simulink model "model"  (R2015a)
settings: Solver=ode45  StartTime=0.0  RelTol=1e-3
values from neighbouring files (symbols this model uses):
  A = [-31.31 0 -2.833e4 2; 0 -10.25 8001 0; 1 -1 0 0; 0 0 0 -100]    [Copy_of_UIE_tracking_main.m]    (also in UIE_main.m = [0 0 1 0; 0 0 0 1; -3 1 -0.4 0.1; 1 -1 0.1 -0.1]; UIE_tracking_main.m = [0 0 1 0; 0 0 0 1; -3 1 -0.4 0.1; 1 -1 0.1 -0.1])
  Af = [-100 0; 0 -100]    [Copy_of_UIE_tracking_main.m]    (also in UIE_main.m; UIE_tracking_main.m)
  B = [28.06 0 0 1; 0 28.06 0 1]'    [Copy_of_UIE_tracking_main.m]    (also in UIE_main.m = [0 0; 0 0; 1 0; 0 1]; UIE_tracking_main.m = [0 0; 0 0; 1 0; 0 1])
  Bd = B    [Copy_of_UIE_tracking_main.m]    (also in UIE_main.m = [0 0 0; 0 0 0; 1 0.5 0.75; 0.5 1 0.75]; UIE_tracking_main.m)
  Bf = [8 0; 0 8]    [Copy_of_UIE_tracking_main.m]    (also in UIE_main.m; UIE_tracking_main.m)
  C = [1 0 0 0;1 0 30 0]    [Copy_of_UIE_tracking_main.m]    (also in UIE_main.m = [1 0 0 0; 0 1 0 0]; UIE_tracking_main.m = [1 0 0 0; 0 1 0 0])
  Cf = [12.5 0; 0 12.5]    [Copy_of_UIE_tracking_main.m]    (also in UIE_main.m; UIE_tracking_main.m)
  Ec = -inv(Rc)*B'*inv(A - B*Kc)'*C'*Qc    [Copy_of_UIE_tracking_main.m]    (also in UIE_main.m; UIE_tracking_main.m)
  Kc = lqr(A + Hc*eye(n), B, C'*Qc*C, Rc)    [Copy_of_UIE_tracking_main.m]    (also in UIE_main.m; UIE_tracking_main.m)
  Kd = pinv(B)*Lt    [Copy_of_UIE_tracking_main.m]    (also in UIE_main.m; UIE_tracking_main.m)
  L = lqr(A'+H*eye(n), C', Qo, Ro)'    [Copy_of_UIE_tracking_main.m]    (also in UIE_main.m; UIE_tracking_main.m)
  Tf = 1e-3    (= 0.001)    [Copy_of_UIE_tracking_main.m]    (also in UIE_main.m; UIE_tracking_main.m)
  x_ini = [0 0 0 0]    [Copy_of_UIE_tracking_main.m]    (also in UIE_main.m = [0 1 0 0]; UIE_tracking_main.m)
  xo_ini = [0 0 0 0]    [Copy_of_UIE_tracking_main.m]    (also in UIE_main.m = [0 1 0 0]; UIE_tracking_main.m)
settings Model: CovSFcnEnable=off  Creator=123  LastModifiedBy=Elca
settings DebuggingCC: UnconnectedInputMsg=none  UnconnectedOutputMsg=none

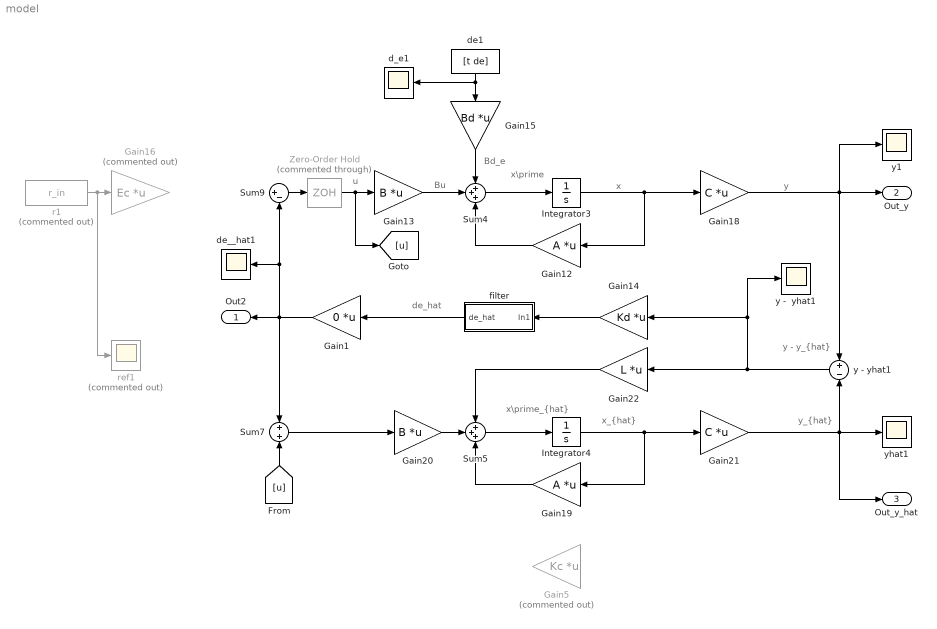
== system model ==
  note: de_hat
  note: Bd_e
  note: Bu
  note: y - y_{hat}
  note: x\prime
  note: x\prime_{hat}
  note: x_{hat}
  note: y_{hat}
  note: x
  note: y
  note: u
  Gain1 : Gain  Gain=0  Multiplication=Matrix(K*u)
  Gain12 : Gain  Gain=A  Multiplication=Matrix(K*u)
  Gain13 : Gain  Gain=B  Multiplication=Matrix(K*u)
  Gain14 : Gain  Gain=Kd  Multiplication=Matrix(K*u)
  Gain15 : Gain  Gain=Bd  Multiplication=Matrix(K*u)
  Gain16 : Gain  Commented=on  Gain=Ec  Multiplication=Matrix(K*u)
  Gain18 : Gain  Gain=C  Multiplication=Matrix(K*u)
  Gain19 : Gain  Gain=A  Multiplication=Matrix(K*u)
  Gain20 : Gain  Gain=B  Multiplication=Matrix(K*u)
  Gain21 : Gain  Gain=C  Multiplication=Matrix(K*u)
  Gain22 : Gain  Gain=L  Multiplication=Matrix(K*u)
  Gain5 : Gain  Commented=on  Gain=Kc  Multiplication=Matrix(K*u)
  Integrator3 : Integrator  InitialCondition=x_ini
  Integrator4 : Integrator  InitialCondition=xo_ini
  Sum4 : Sum  Inputs=+++
  Sum5 : Sum  Inputs=+++
  Sum7 : Sum  Inputs=+|+
  Sum9 : Sum  Inputs=|+-
  Zero-Order Hold : ZeroOrderHold  Commented=through  SampleTime=Tf
  d_e1 : Scope
      settings: TickLabels=on  ShowLegends=on  SaveName=ScopeData6  ScrollMode=on
  de1 : FromWorkspace  VariableName=[t de]  SampleTime=0
  de__hat1 : Scope
      settings: TickLabels=on  ShowLegends=on  SaveName=ScopeData7  ScrollMode=on
  filter : Subsystem
  r1 : FromWorkspace  Commented=on  VariableName=r_in  SampleTime=Tf
  ref1 : Scope  Commented=on
      settings: TickLabels=on  YMin=0  YMax=550000  SaveName=ScopeData11  ScrollMode=on
  y -  yhat1 : Scope
      settings: TickLabels=on  ShowLegends=on  SaveName=ScopeData8  ScrollMode=on
  y - yhat1 : Sum  Inputs=+-
  y1 : Scope
      settings: TickLabels=on  YMin=-0.8  YMax=1  SaveName=ScopeData9  ScrollMode=on
  yhat1 : Scope
      settings: TickLabels=on  ShowLegends=on  SaveName=ScopeData10  ScrollMode=on
  Out2 : Outport
  Out_y : Outport  Port=2
  Out_y_hat : Outport  Port=3
  wires:
  Sum4/1 -> Integrator3/1
  Integrator3/1 -> Gain12/1, Gain18/1
  Sum5/1 -> Integrator4/1
  Integrator4/1 -> Gain19/1, Gain21/1
  Gain19/1 -> Sum5/3
  Gain20/1 -> Sum5/2
  y - yhat1/1 -> Gain22/1, Gain14/1, y -  yhat1/1
  Gain22/1 -> Sum5/1
  Gain21/1 -> Out_y_hat/1, y - yhat1/2, yhat1/1
  Gain18/1 -> y - yhat1/1, y1/1, Out_y/1
  de1/1 -> Gain15/1, d_e1/1
  Gain12/1 -> Sum4/3
  Gain13/1 -> Sum4/2
  [u] -> Sum7/2
  Zero-Order Hold/1 -> Gain13/1, [u]
  filter/1(de_hat) -> Gain1/1
  Gain14/1 -> filter/1(In1)
  Gain15/1 -> Sum4/1
  r1/1 -> ref1/1, Gain16/1
  Sum9/1 -> Zero-Order Hold/1
  Sum7/1 -> Gain20/1
  Gain1/1 -> Sum9/2, de__hat1/1, Sum7/1, Out2/1

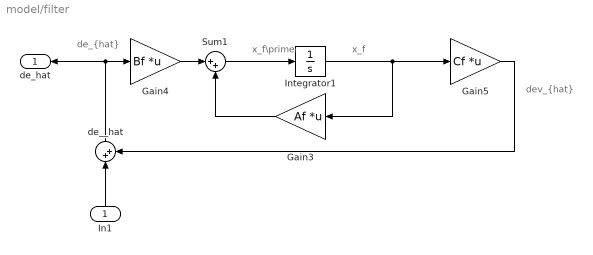
== system model/filter ==
  note: x_f\prime
  note: x_f
  note: dev_{hat}
  note: de_{hat}
  In1 : Inport
  Gain3 : Gain  Gain=Af  Multiplication=Matrix(K*u)
  Gain4 : Gain  Gain=Bf  Multiplication=Matrix(K*u)
  Gain5 : Gain  Gain=Cf  Multiplication=Matrix(K*u)
  Integrator1 : Integrator
  Sum1 : Sum  Inputs=|++
  de__hat : Sum  Inputs=|++
  de_hat : Outport
  wires:
  Gain4/1 -> Sum1/1
  Sum1/1 -> Integrator1/1
  Integrator1/1 -> Gain3/1, Gain5/1
  Gain3/1 -> Sum1/2
  de__hat/1 -> de_hat/1, Gain4/1
  Gain5/1 -> de__hat/2
  In1/1 -> de__hat/1
